simulink model "hw_WiFi"  (R2020b)
settings: Solver=FixedStepAuto  StartTime=0.0  StopTime=inf  RelTol=1e-3  EnableMultiTasking=on
libraries: arduinowifilib x5, simulink x1
settings Model: SILPILModeSetting=veronly  ExtModeTrigDuration=2  Creator=Callum  LastModifiedBy=Callum
settings OptimizationCC: EnhancedBackFolding=on  PassReuseOutputArgsAs=Individual arguments  ZeroExternalMemoryAtStartup=off  ZeroInternalMemoryAtStartup=off  MaxStackSize=64  OptimizeBlockOrder=speed  DifferentSizesBufferReuse=on  OptimizationCustomize=off  EfficientTunableParamExpr=on
settings DebuggingCC: ParameterTunabilityLossMsg=error
settings HardwareCC: ProdBitPerPointer=32  ProdBitPerSizeT=32  ProdBitPerPtrDiffT=32  ProdLargestAtomicInteger=Long  ProdLargestAtomicFloat=Double  ProdWordSize=32  ProdHWDeviceType=ARM Compatible->ARM Cortex  UseEmbeddedCoderFeatures=off  UseSimulinkCoderFeatures=off
settings SFSimCC: MATLABDynamicMemAlloc=off
settings RTWCC: Description=Embedded Coder  SystemTargetFile=ert.tlc  HardwareBoard=Arduino Nano 33 IoT  TemplateMakefile=ert_default_tmf  Toolchain=Arduino ARM  BuildConfiguration=Faster Runs
settings CodeAppCC: ForceParamTrailComments=on  IgnoreCustomStorageClasses=off  OperatorAnnotations=on  SimulinkDataObjDesc=on  SFDataObjDesc=on  InsertBlockDesc=on
settings ERTTargetCC: SupportContinuousTime=on  SupportNonInlinedSFcns=on  SupportVariableSizeSignals=on  ExtModeTransport=3  ExtModeStaticAllocSize=8192  ExtModeMexFile=ext_xcp  ExtModeIntrfLevel=Level2 - Open

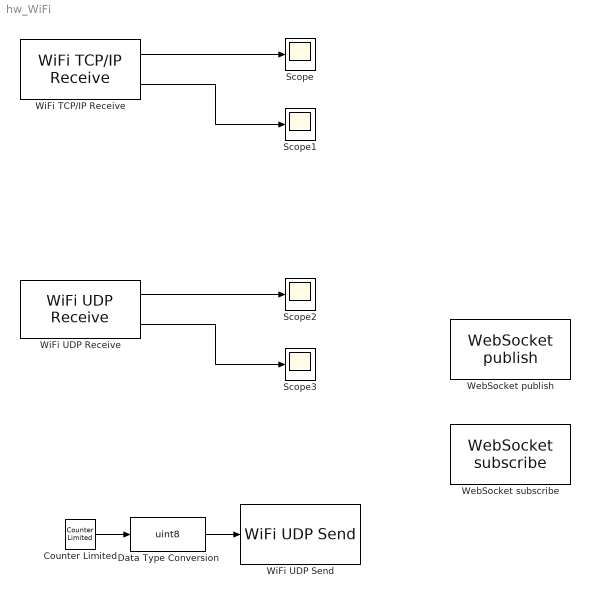
== system hw_WiFi ==
  Counter Limited : simulink/Sources/Counter Limited  uplimit=20  tsamp=-1
  Data Type Conversion : DataTypeConversion  OutDataTypeStr=uint8
  Scope{,1..3} (4 alike) : Scope
  WebSocket publish : arduinowifilib/WebSocket publish  Port=9000  NumberOfSignals=2
      settings: SourceProductBaseCode=ARDUINO
  WebSocket subscribe : arduinowifilib/WebSocket subscribe  Port=9000  OutputCfg=Mask Dialog  numSignals=1  Dsize1=1  Dtype1=double  Dsize2=1  Dtype2=double  Dsize3=1  Dtype3=double  Dsize4=1  Dtype4=double  Dsize5=1  Dtype5=double  Dsize6=1  Dtype6=double  Dsize7=1  Dtype7=double  Dsize8=1  Dtype8=double  Dsize9=1  Dtype9=double  Dsize10=1  Dtype10=double  Sampletime=0.1
      settings: SourceProductBaseCode=ARDUINO
  WiFi TCP/IP Receive : arduinowifilib/WiFi TCP//IP Receive  Mode_=Server  serverport=25000  RemoteAddr_=192.168.1.2  RemoteServerPort_=25000  DataType_=uint8  DataSize_=1  SampleTime_=0.1  remoteipoctet1=192  remoteipoctet2=168  remoteipoctet3=1  remoteipoctet4=2  wifiTCPServerIndex=0  wifiTCPClientIndex=0  blockPlatform=ARDUINO  isARMArch=true  SimulateUsing=Code generation  BlockingMode_=off  BlockTimeout_=0.1
      settings: SourceProductBaseCode=ARDUINO
  WiFi UDP Receive : arduinowifilib/WiFi UDP Receive  localport=50001  DataType=uint8  DataLength=14  SampleTime_=1  wifiUDPIndex=0  blockPlatform=ARDUINO  isARMArch=true
      settings: SourceProductBaseCode=ARDUINO
  WiFi UDP Send : arduinowifilib/WiFi UDP Send  remoteIPOctetString=192.168.0.14  remoteport=50002  localport=50003  remoteipoctet1=192  remoteipoctet2=168  remoteipoctet3=0  remoteipoctet4=14  wifiUDPIndex=1  blockPlatform=ARDUINO  isARMArch=true
      settings: SourceProductBaseCode=ARDUINO
  wires:
  WiFi TCP/IP Receive/1 -> Scope/1
  WiFi TCP/IP Receive/2 -> Scope1/1
  WiFi UDP Receive/2 -> Scope3/1
  WiFi UDP Receive/1 -> Scope2/1
  Counter Limited/1 -> Data Type Conversion/1
  Data Type Conversion/1 -> WiFi UDP Send/1
